simulink model "Andrej_Klein_zadanie1C_S_v2021a"  (R2021a)
settings: Solver=VariableStepAuto  StartTime=0.0  StopTime=10  RelTol=1e-3
model workspace (MAT data in the model file):
  Al = 3
  a1 = -0.47
  b1 = -3.32
  c1 = -0.05
  d1 = -0.13
  e1 = 2.5
  v = 0.12
settings Model: OrderedModelArguments=off  Creator=hwswi  LastModifiedBy=hwswi
settings DebuggingCC: UnconnectedInputMsg=none  UnconnectedOutputMsg=none  UnconnectedLineMsg=none
settings ModelReferenceCC: EnableRefExpFcnMdlSchedulingChecks=off
settings RTWCC: Description=Generic Real-Time Target  DLArmComputeVersion=20.02.1

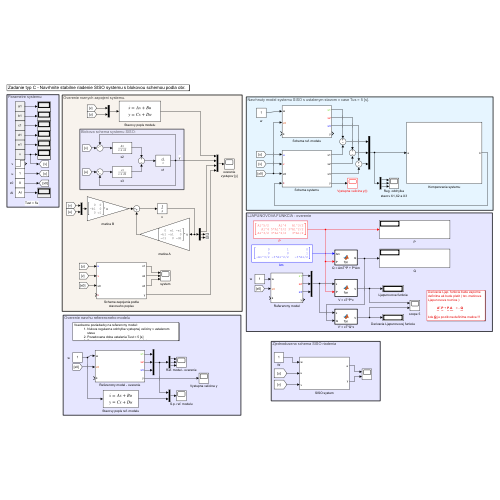
[thumbnail: Simulink's stored preview of the top-level diagram]
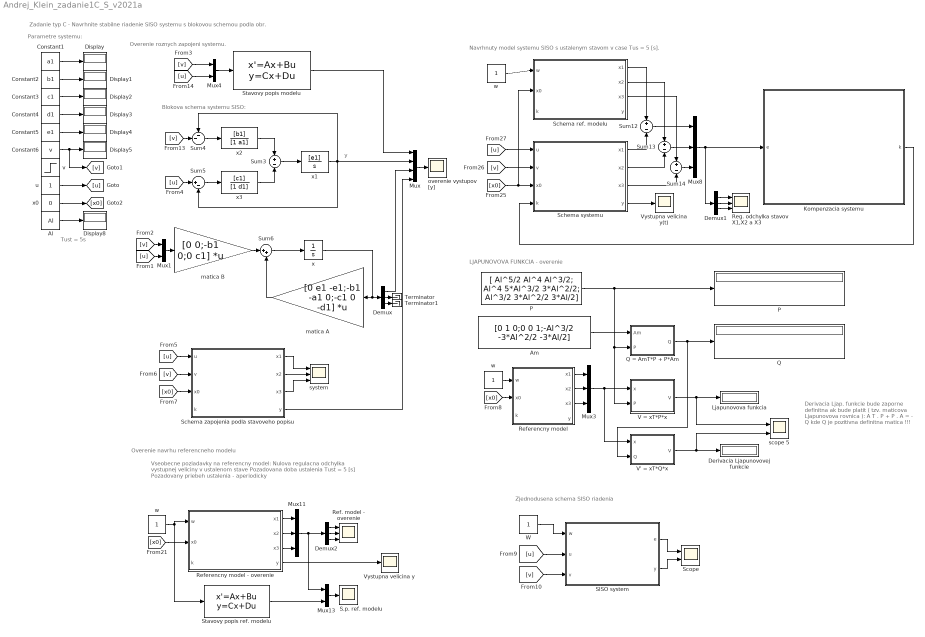
== system Andrej_Klein_zadanie1C_S_v2021a ==
  note: Zjednodusena schema SISO riadenia
  note: Overenie navrhu referencneho modelu
  note: Zadanie typ C - Navrhnite stabilne riadenie SISO systemu s blokovou schemou podla obr.
  note: LJAPUNOVOVA FUNKCIA - overenie
  note: Navrhnuty model systemu SISO s ustalenym stavom v case Tus = 5 [s].
  note: y
  note: Overenie roznych zapojeni systemu.
  note: Blokova schema systemu SISO:
  note: Parametre systemu:
  note: Tust = 5s
  note: Vseobecne poziadavky na referencny model:
      | Nulova regulacna odchylka vystupnej veliciny v ustalenom stave
      | Pozadovana doba ustalenia Tust = 5 [s]
      | Pozadovany priebeh ustalenia - aperiodicky
  note: Derivacia Ljap. funkcie bude zaporne definitna ak bude platit ( tzv. maticova Ljapunovova rovnica ):
      |
      | A T . P + P . A = - Q
      |
      | kde Q je pozitivna definitna matica !!!
  " w " : Constant
  Al : Constant  Value=Al
  "Am  " : Constant  Value=[0 1 0;0 0 1;-Al^3/2 -3*Al^2/2 -3*Al/2]
  Constant1 : Constant  Value=a1
  Constant2 : Constant  Value=b1
  Constant3 : Constant  Value=c1
  Constant4 : Constant  Value=d1
  Constant5 : Constant  Value=e1
  Constant6 : Constant  Value=v
  Demux : Demux  Outputs=3
  Demux1 : Demux  Outputs=3
  Demux2 : Demux  Outputs=3
  Derivacia Ljapunovovej funkcie : Display
  Display{,1..5,8} (7 alike) : Display
  Kompenzacia systemu : Subsystem
  Ljapunovova funkcia : Display
  Mux : Mux
  Mux1 : Mux  Inputs=2
  Mux11 : Mux  Inputs=3
  Mux13 : Mux  Inputs=2
  Mux3 : Mux  Inputs=3
  Mux4 : Mux  Inputs=2
  Mux8 : Mux  Inputs=3
  P : Display
  "P  " : Constant  Value="[ Al^5/2  Al^4  Al^3/2; Al^4 5*Al^3/2 3*Al^2/2; Al^3/2 3*Al^2/2 3*Al/2]"
  Q : Display
  Q = AmT*P + P*Am : MATLAB Function  TreatAsAtomicUnit=on
  Ref. model - overenie : Scope  NumInputPorts=3
  Referencny model : Subsystem
  Referencny model - overenie : Subsystem
  Reg. odchylka stavov X1,X2 a X3 : Scope  NumInputPorts=3
  S.p. ref. modelu : Scope
  SISO system : Subsystem
  Schema ref. modelu : Subsystem
  Schema systemu : Subsystem
  Schema zapojenia podla stavoveho popisu : Subsystem
  Scope : Scope  NumInputPorts=2
  Stavovy popis modelu : StateSpace  A=[0 e1 -e1;-b1 -a1 0;-c1 0 -d1]  B=[0 0;-b1 0;0 c1]  C=[1 0 0]  D=[0 0]  InitialCondition=0
  Stavovy popis ref. modelu : StateSpace  A=[0 1 0;0 0 1;-Al^3/2 -3*Al^2/2 -3*Al/2]  B=[0;0;Al^3/2]  C=[1 0 0;0 1 0;0 0 1]  D=[0;0;0]  InitialCondition=0
  Sum{3,12..14} (4 alike) : Sum  Inputs=+-
  Sum4 : Sum  Inputs=--|
  Sum5 : Sum  Inputs=|+-
  Sum6 : Sum  Inputs=|++
  Terminator : Terminator
  Terminator1 : Terminator
  V = xT*P*x : MATLAB Function  TreatAsAtomicUnit=on
  V' = xT*Q*x : MATLAB Function  TreatAsAtomicUnit=on
  Vystupna velicina y : Scope
  Vystupna velicina y(t) : Scope
  W : Constant
  matica A : Gain  Gain=[0 e1 -e1;-b1 -a1 0;-c1 0 -d1]  Multiplication=Matrix(K*u)
  matica B : Gain  Gain=[0 0;-b1 0;0 c1]  Multiplication=Matrix(K*u)
  overenie vystupov [y] : Scope
  scope 5 : Scope  NumInputPorts=2
  system : Scope  NumInputPorts=3
  u : Constant
  v : Step  Before=v  After=5*v  SampleTime=0
  w : Constant
  "w " : Constant
  x : Integrator
  x0 : Constant  Value=0
  x1 : TransferFcn  Numerator=[e1]  Denominator=[1 0]
  x2 : TransferFcn  Numerator=[b1]  Denominator=[1 a1]
  x3 : TransferFcn  Numerator=[c1]  Denominator=[1 d1]
  wires:
  Mux13/1 -> S.p. ref. modelu/1
  Referencny model - overenie/1(x1) -> Mux11/1
  Referencny model - overenie/2(x2) -> Mux11/2
  Mux11/1 -> Demux2/1, Mux13/1
  Referencny model - overenie/3(x3) -> Mux11/3
  [x0] -> Referencny model - overenie/2(x0)
  "w "/1 -> Stavovy popis ref. modelu/1, Referencny model - overenie/1(w)
  Stavovy popis ref. modelu/1 -> Mux13/2
  Kompenzacia systemu/1(k) -> Schema systemu/4(k)
  Sum12/1 -> Mux8/1
  Sum13/1 -> Mux8/2
  Mux8/1 -> Kompenzacia systemu/1(e), Demux1/1
  Schema systemu/3(x3) -> Sum14/2
  Schema systemu/1(x1) -> Sum12/2
  Schema ref. modelu/1(x1) -> Sum12/1
  Sum14/1 -> Mux8/3
  Schema ref. modelu/2(x2) -> Sum13/1
  [u] -> Schema systemu/1(u)
  [x0] -> Schema ref. modelu/2(x0), Schema systemu/3(x0)
  Schema ref. modelu/3(x3) -> Sum14/1
  [v] -> Schema systemu/2(v)
  Schema systemu/2(x2) -> Sum13/2
  w/1 -> Schema ref. modelu/1(w)
  Sum5/1 -> x3/1
  [u] -> Mux4/2
  Stavovy popis modelu/1 -> Mux/1
  [v] -> Mux4/1
  [u] -> Sum5/1
  [v] -> Sum4/2
  Mux/1 -> overenie vystupov [y]/1
  Mux4/1 -> Stavovy popis modelu/1
  Sum4/1 -> x2/1
  x3/1 -> Sum3/2
  Sum3/1 -> x1/1
  x1/1 -> Sum5/2, Mux/2, Sum4/1
  x2/1 -> Sum3/1
  Constant4/1 -> Display3/1
  Constant5/1 -> Display4/1
  x0/1 -> [x0]
  Al/1 -> Display8/1
  Constant6/1 -> [v], Display5/1
  u/1 -> [u]
  Constant3/1 -> Display2/1
  Constant1/1 -> Display/1
  Constant2/1 -> Display1/1
  x/1 -> Demux/1, matica A/1
  Demux/3 -> Terminator1/1
  matica A/1 -> Sum6/2
  Mux1/1 -> matica B/1
  matica B/1 -> Sum6/1
  Sum6/1 -> x/1
  Demux/2 -> Terminator/1
  [v] -> Mux1/1
  [u] -> Mux1/2
  Demux/1 -> Mux/3
  Schema zapojenia podla stavoveho popisu/4(y) -> Mux/4
  [u] -> Schema zapojenia podla stavoveho popisu/1(u)
  [v] -> Schema zapojenia podla stavoveho popisu/2(v)
  [x0] -> Schema zapojenia podla stavoveho popisu/3(x0)
  Schema zapojenia podla stavoveho popisu/1(x1) -> system/1
  Schema zapojenia podla stavoveho popisu/2(x2) -> system/2
  Schema zapojenia podla stavoveho popisu/3(x3) -> system/3
  "P  "/1 -> P/1, V = xT*P*x/2(P), Q = AmT*P + P*Am/2(P)
  Q = AmT*P + P*Am/1(Q) -> Q/1, V' = xT*Q*x/2(Q)
  " w "/1 -> Referencny model/1(w)
  Referencny model/1(x1) -> Mux3/1
  Referencny model/2(x2) -> Mux3/2
  Referencny model/3(x3) -> Mux3/3
  [x0] -> Referencny model/2(x0)
  Mux3/1 -> V' = xT*Q*x/1(x), V = xT*P*x/1(x)
  "Am  "/1 -> Q = AmT*P + P*Am/1(Am)
  V' = xT*Q*x/1(V) -> Derivacia Ljapunovovej funkcie/1, scope 5/2
  V = xT*P*x/1(V) -> scope 5/1, Ljapunovova funkcia/1
  W/1 -> SISO system/1(w)
  [u] -> SISO system/2(u)
  [v] -> SISO system/3(v)
  SISO system/1(e) -> Scope/1
  SISO system/2(y) -> Scope/2
  Schema systemu/4(y) -> Vystupna velicina y(t)/1
  Demux1/1 -> Reg. odchylka stavov X1,X2 a X3/1
  Demux1/2 -> Reg. odchylka stavov X1,X2 a X3/2
  Demux1/3 -> Reg. odchylka stavov X1,X2 a X3/3
  Referencny model - overenie/4(y) -> Vystupna velicina y/1
  Demux2/2 -> Ref. model - overenie/2
  Demux2/1 -> Ref. model - overenie/1
  Demux2/3 -> Ref. model - overenie/3

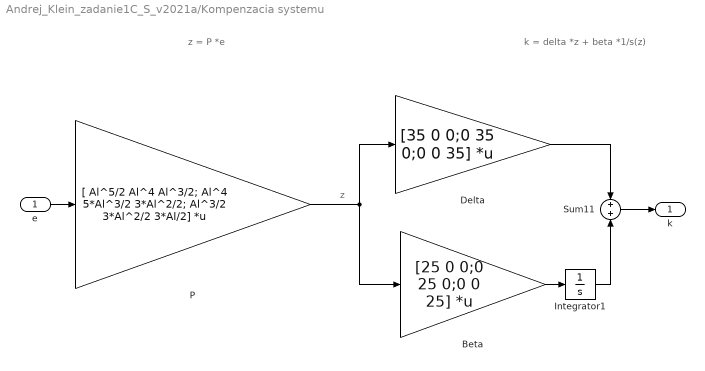
== system Andrej_Klein_zadanie1C_S_v2021a/Kompenzacia systemu ==
  note: z
  note: k = delta *z + beta *1/s(z)
  note: z = P *e
  e : Inport
  Beta : Gain  Gain=[25 0 0;0 25 0;0 0 25]  Multiplication=Matrix(K*u)
  Delta : Gain  Gain=[35 0 0;0 35 0;0 0 35]  Multiplication=Matrix(K*u)
  Integrator1 : Integrator
  P : Gain  Gain="[ Al^5/2  Al^4  Al^3/2; Al^4 5*Al^3/2 3*Al^2/2; Al^3/2 3*Al^2/2 3*Al/2]"  Multiplication=Matrix(K*u)
  Sum11 : Sum
  k : Outport
  wires:
  Integrator1/1 -> Sum11/2
  Beta/1 -> Integrator1/1
  Sum11/1 -> k/1
  e/1 -> P/1
  Delta/1 -> Sum11/1
  P/1 -> Beta/1, Delta/1

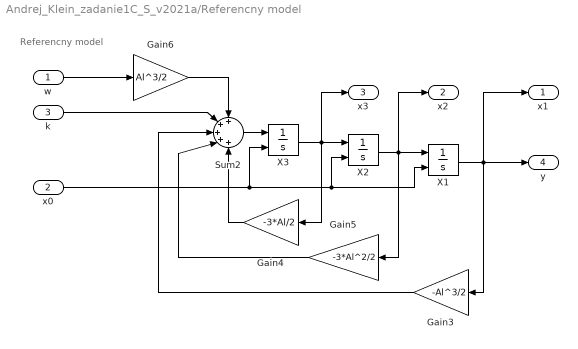
== system Andrej_Klein_zadanie1C_S_v2021a/Referencny model ==
  note: Referencny model
  w : Inport
  x0 : Inport  Port=2
  k : Inport  Port=3
  Gain3 : Gain  Gain=-Al^3/2
  Gain4 : Gain  Gain=-3*Al/2
  Gain5 : Gain  Gain=-3*Al^2/2
  Gain6 : Gain  Gain=Al^3/2
  Sum2 : Sum  Inputs=+++++
  X1 : Integrator  InitialConditionSource=external
  X2 : Integrator  InitialConditionSource=external
  X3 : Integrator  InitialConditionSource=external
  x1 : Outport
  x2 : Outport  Port=2
  x3 : Outport  Port=3
  y : Outport  Port=4
  wires:
  k/1 -> Sum2/2
  Gain6/1 -> Sum2/1
  x0/1 -> X3/2, X2/2, X1/2
  Gain3/1 -> Sum2/3
  w/1 -> Gain6/1
  X2/1 -> x2/1, X1/1, Gain5/1
  X3/1 -> x3/1, X2/1, Gain4/1
  Gain4/1 -> Sum2/5
  X1/1 -> y/1, x1/1, Gain3/1
  Sum2/1 -> X3/1
  Gain5/1 -> Sum2/4

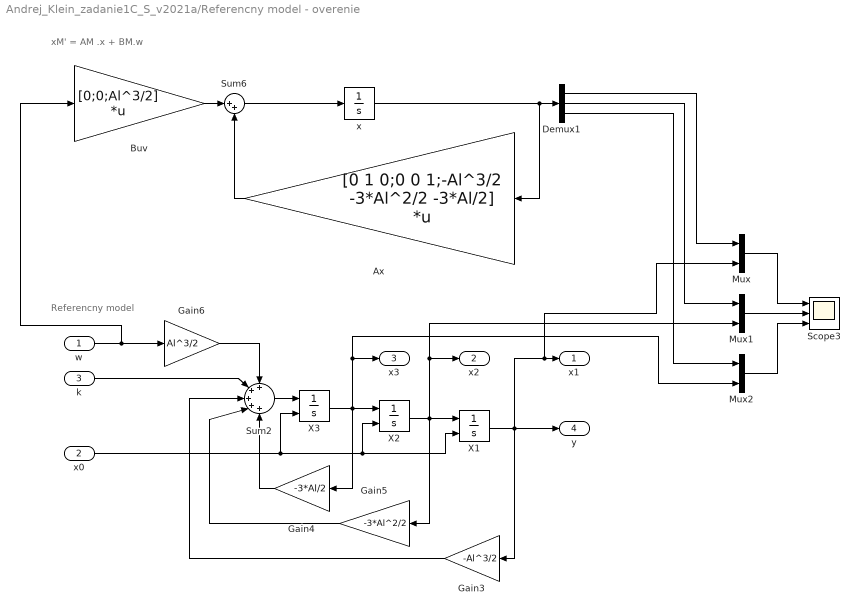
== system Andrej_Klein_zadanie1C_S_v2021a/Referencny model - overenie ==
  note: Referencny model
  note: xM' = AM .x + BM.w
  w : Inport
  x0 : Inport  Port=2
  k : Inport  Port=3
  Ax : Gain  Gain=[0 1 0;0 0 1;-Al^3/2 -3*Al^2/2 -3*Al/2]  Multiplication=Matrix(K*u)
  Buv : Gain  Gain=[0;0;Al^3/2]  Multiplication=Matrix(K*u)
  Demux1 : Demux  Outputs=3
  Gain3 : Gain  Gain=-Al^3/2
  Gain4 : Gain  Gain=-3*Al/2
  Gain5 : Gain  Gain=-3*Al^2/2
  Gain6 : Gain  Gain=Al^3/2
  Mux : Mux  Inputs=2
  Mux1 : Mux  Inputs=2
  Mux2 : Mux  Inputs=2
  Scope3 : Scope  NumInputPorts=3
  Sum2 : Sum  Inputs=+++++
  Sum6 : Sum  Inputs=|++
  X1 : Integrator  InitialConditionSource=external
  X2 : Integrator  InitialConditionSource=external
  X3 : Integrator  InitialConditionSource=external
  x : Integrator
  x1 : Outport
  x2 : Outport  Port=2
  x3 : Outport  Port=3
  y : Outport  Port=4
  wires:
  Gain5/1 -> Sum2/4
  Sum2/1 -> X3/1
  Demux1/2 -> Mux1/1
  X1/1 -> y/1, Mux/2, x1/1, Gain3/1
  X2/1 -> Mux1/2, x2/1, X1/1, Gain5/1
  Mux2/1 -> Scope3/3
  Mux1/1 -> Scope3/2
  Mux/1 -> Scope3/1
  Gain4/1 -> Sum2/5
  w/1 -> Gain6/1, Buv/1
  Demux1/3 -> Mux2/1
  x/1 -> Demux1/1, Ax/1
  Demux1/1 -> Mux/1
  Buv/1 -> Sum6/1
  Gain3/1 -> Sum2/3
  Sum6/1 -> x/1
  X3/1 -> x3/1, Mux2/2, X2/1, Gain4/1
  x0/1 -> X3/2, X2/2, X1/2
  Gain6/1 -> Sum2/1
  k/1 -> Sum2/2
  Ax/1 -> Sum6/2

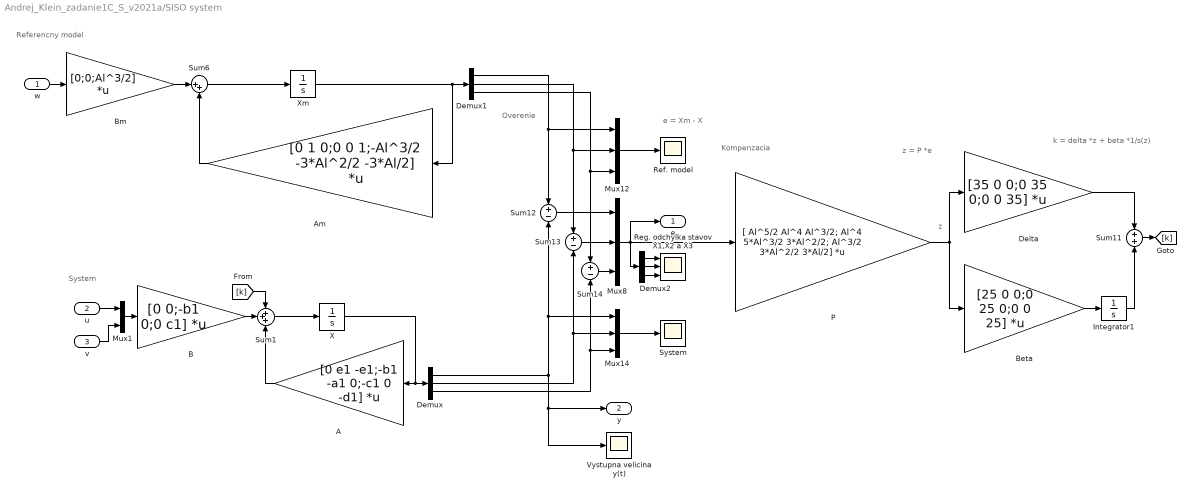
== system Andrej_Klein_zadanie1C_S_v2021a/SISO system ==
  note: e = Xm - X
  note: Overenie
  note: Kompenzacia
  note: Referencny model
  note: System
  note: z
  note: k = delta *z + beta *1/s(z)
  note: z = P *e
  w : Inport
  u : Inport  Port=2
  v : Inport  Port=3
  A : Gain  Gain=[0 e1 -e1;-b1 -a1 0;-c1 0 -d1]  Multiplication=Matrix(K*u)
  Am : Gain  Gain=[0 1 0;0 0 1;-Al^3/2 -3*Al^2/2 -3*Al/2]  Multiplication=Matrix(K*u)
  "B " : Gain  Gain=[0 0;-b1 0;0 c1]  Multiplication=Matrix(K*u)
  Beta : Gain  Gain=[25 0 0;0 25 0;0 0 25]  Multiplication=Matrix(K*u)
  Bm : Gain  Gain=[0;0;Al^3/2]  Multiplication=Matrix(K*u)
  Delta : Gain  Gain=[35 0 0;0 35 0;0 0 35]  Multiplication=Matrix(K*u)
  Demux : Demux  Outputs=3
  Demux1 : Demux  Outputs=3
  Demux2 : Demux  Outputs=3
  Integrator1 : Integrator
  Mux1 : Mux  Inputs=2
  Mux12 : Mux  Inputs=3
  Mux14 : Mux  Inputs=3
  Mux8 : Mux  Inputs=3
  P : Gain  Gain="[ Al^5/2  Al^4  Al^3/2; Al^4 5*Al^3/2 3*Al^2/2; Al^3/2 3*Al^2/2 3*Al/2]"  Multiplication=Matrix(K*u)
  Ref. model : Scope
  Reg. odchylka stavov X1,X2 a X3 : Scope  NumInputPorts=3
  Sum1 : Sum  Inputs=+++
  Sum11 : Sum
  Sum12 : Sum  Inputs=+-
  Sum13 : Sum  Inputs=+-
  Sum14 : Sum  Inputs=+-
  Sum6 : Sum  Inputs=|++
  System : Scope
  Vystupna velicina y(t) : Scope
  X : Integrator
  Xm : Integrator
  e : Outport
  y : Outport  Port=2
  wires:
  Am/1 -> Sum6/2
  Sum6/1 -> Xm/1
  Bm/1 -> Sum6/1
  Xm/1 -> Am/1, Demux1/1
  w/1 -> Bm/1
  "B "/1 -> Sum1/2
  Mux1/1 -> "B "/1
  X/1 -> Demux/1, A/1
  A/1 -> Sum1/3
  Sum1/1 -> X/1
  Integrator1/1 -> Sum11/2
  Beta/1 -> Integrator1/1
  Delta/1 -> Sum11/1
  P/1 -> Beta/1, Delta/1
  Sum14/1 -> Mux8/3
  Demux1/3 -> Sum14/1, Mux12/3
  Demux/1 -> Vystupna velicina y(t)/1, y/1, Sum12/2, Mux14/1
  Demux1/1 -> Sum12/1, Mux12/1
  Mux12/1 -> Ref. model/1
  Demux/2 -> Sum13/2, Mux14/2
  Demux/3 -> Sum14/2, Mux14/3
  Mux8/1 -> e/1, Demux2/1, P/1
  Sum13/1 -> Mux8/2
  Demux1/2 -> Sum13/1, Mux12/2
  Sum12/1 -> Mux8/1
  Mux14/1 -> System/1
  Sum11/1 -> [k]
  [k] -> Sum1/1
  u/1 -> Mux1/1
  v/1 -> Mux1/2
  Demux2/3 -> Reg. odchylka stavov X1,X2 a X3/3
  Demux2/2 -> Reg. odchylka stavov X1,X2 a X3/2
  Demux2/1 -> Reg. odchylka stavov X1,X2 a X3/1

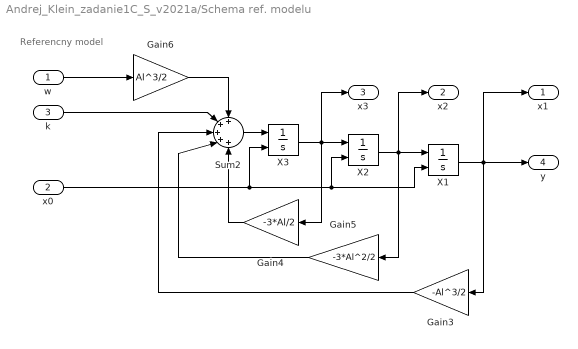
== system Andrej_Klein_zadanie1C_S_v2021a/Schema ref. modelu ==
  note: Referencny model
  w : Inport
  x0 : Inport  Port=2
  k : Inport  Port=3
  Gain3 : Gain  Gain=-Al^3/2
  Gain4 : Gain  Gain=-3*Al/2
  Gain5 : Gain  Gain=-3*Al^2/2
  Gain6 : Gain  Gain=Al^3/2
  Sum2 : Sum  Inputs=+++++
  X1 : Integrator  InitialConditionSource=external
  X2 : Integrator  InitialConditionSource=external
  X3 : Integrator  InitialConditionSource=external
  x1 : Outport
  x2 : Outport  Port=2
  x3 : Outport  Port=3
  y : Outport  Port=4
  wires:
  Gain5/1 -> Sum2/4
  X1/1 -> y/1, x1/1, Gain3/1
  X2/1 -> x2/1, X1/1, Gain5/1
  Sum2/1 -> X3/1
  Gain4/1 -> Sum2/5
  x0/1 -> X3/2, X2/2, X1/2
  Gain3/1 -> Sum2/3
  Gain6/1 -> Sum2/1
  X3/1 -> x3/1, X2/1, Gain4/1
  w/1 -> Gain6/1
  k/1 -> Sum2/2

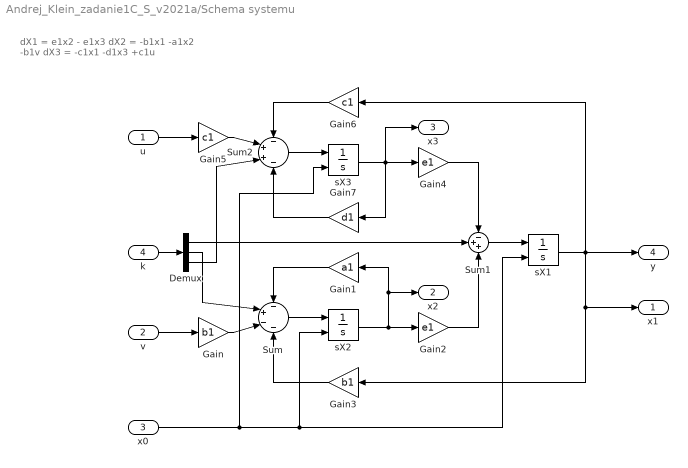
== system Andrej_Klein_zadanie1C_S_v2021a/Schema systemu ==
  note: dX1 = e1x2 - e1x3
      | dX2 = -b1x1 -a1x2 -b1v
      | dX3 = -c1x1 -d1x3 +c1u
  u : Inport
  v : Inport  Port=2
  x0 : Inport  Port=3
  k : Inport  Port=4
  Demux : Demux  Outputs=3
  Gain : Gain  Gain=b1
  Gain1 : Gain  Gain=a1
  Gain2 : Gain  Gain=e1
  Gain3 : Gain  Gain=b1
  Gain4 : Gain  Gain=e1
  Gain5 : Gain  Gain=c1
  Gain6 : Gain  Gain=c1
  Gain7 : Gain  Gain=d1
  Sum : Sum  Inputs=-+--
  Sum1 : Sum  Inputs=-++
  Sum2 : Sum  Inputs=-++-
  sX1 : Integrator  InitialConditionSource=external
  sX2 : Integrator  InitialConditionSource=external
  sX3 : Integrator  InitialConditionSource=external
  x1 : Outport
  x2 : Outport  Port=2
  x3 : Outport  Port=3
  y : Outport  Port=4
  wires:
  Demux/3 -> Sum2/3
  Demux/2 -> Sum/2
  Demux/1 -> Sum1/2
  k/1 -> Demux/1
  Gain7/1 -> Sum2/4
  Gain6/1 -> Sum2/1
  Gain5/1 -> Sum2/2
  u/1 -> Gain5/1
  Gain4/1 -> Sum1/1
  Sum2/1 -> sX3/1
  sX3/1 -> Gain7/1, x3/1, Gain4/1
  sX1/1 -> Gain6/1, y/1, Gain3/1, x1/1
  Sum1/1 -> sX1/1
  Gain2/1 -> Sum1/3
  Gain3/1 -> Sum/4
  sX2/1 -> x2/1, Gain1/1, Gain2/1
  Sum/1 -> sX2/1
  Gain1/1 -> Sum/1
  v/1 -> Gain/1
  Gain/1 -> Sum/3
  x0/1 -> sX3/2, sX2/2, sX1/2

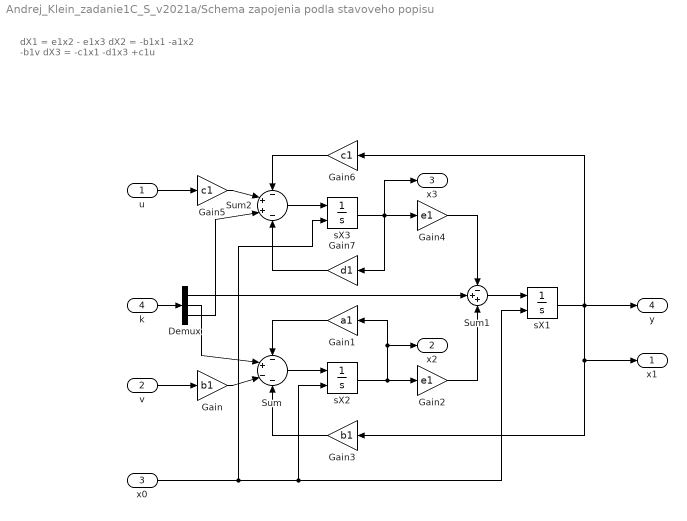
== system Andrej_Klein_zadanie1C_S_v2021a/Schema zapojenia podla stavoveho popisu ==
  note: dX1 = e1x2 - e1x3
      | dX2 = -b1x1 -a1x2 -b1v
      | dX3 = -c1x1 -d1x3 +c1u
  u : Inport
  v : Inport  Port=2
  x0 : Inport  Port=3
  k : Inport  Port=4
  Demux : Demux  Outputs=3
  Gain : Gain  Gain=b1
  Gain1 : Gain  Gain=a1
  Gain2 : Gain  Gain=e1
  Gain3 : Gain  Gain=b1
  Gain4 : Gain  Gain=e1
  Gain5 : Gain  Gain=c1
  Gain6 : Gain  Gain=c1
  Gain7 : Gain  Gain=d1
  Sum : Sum  Inputs=-+--
  Sum1 : Sum  Inputs=-++
  Sum2 : Sum  Inputs=-++-
  sX1 : Integrator  InitialConditionSource=external
  sX2 : Integrator  InitialConditionSource=external
  sX3 : Integrator  InitialConditionSource=external
  x1 : Outport
  x2 : Outport  Port=2
  x3 : Outport  Port=3
  y : Outport  Port=4
  wires:
  x0/1 -> sX1/2, sX2/2, sX3/2
  Gain/1 -> Sum/3
  v/1 -> Gain/1
  Gain1/1 -> Sum/1
  Sum/1 -> sX2/1
  sX2/1 -> Gain2/1, Gain1/1, x2/1
  Gain3/1 -> Sum/4
  Gain2/1 -> Sum1/3
  Sum1/1 -> sX1/1
  sX1/1 -> x1/1, Gain3/1, y/1, Gain6/1
  sX3/1 -> Gain4/1, x3/1, Gain7/1
  Sum2/1 -> sX3/1
  Gain4/1 -> Sum1/1
  u/1 -> Gain5/1
  Gain5/1 -> Sum2/2
  Gain6/1 -> Sum2/1
  Gain7/1 -> Sum2/4
  k/1 -> Demux/1
  Demux/1 -> Sum1/2
  Demux/2 -> Sum/2
  Demux/3 -> Sum2/3

== matlab function Andrej_Klein_zadanie1C_S_v2021a/V' = xT*Q*x ==
  data: x input; V output; Q input
function V = fcn(x,Q)
V = x'*Q*x;

== matlab function Andrej_Klein_zadanie1C_S_v2021a/Q = AmT*P + P*Am ==
  data: Am input; Q output; P input
function Q = fcn(Am,P)
Q = ((Am'*P)+(P*Am));

== matlab function Andrej_Klein_zadanie1C_S_v2021a/V = xT*P*x ==
  data: x input; V output; P input
function V = fcn(x,P)
V = x'*P*x;
